simulink model "arch_logical"  (R2023b)
settings: Solver=VariableStepAuto  StartTime=0.0  StopTime=2  RelTol=1e-3
model workspace (MAT data in the model file):
  pendulum_type = Simulink.Parameter
  pendulum_type.Value = 1
  pendulum_type.DataType = 'uint8'
  pendulum_type.DocUnits = '1'
  pendulum_type.Complexity = 'real'
  pendulum_type.Dimensions = [1 1]
undefined symbols (not defined in the file): pendulum_mass
settings Model: DataDictionary=data_interface.sldd  Creator=upattacini  LastModifiedBy=upattacini
settings DataIOCC: SaveOutput=off  DSMLogging=off  SaveTime=off  ReturnWorkspaceOutputs=off
settings ModelReferenceCC: ModelReferenceNumInstancesAllowed=Single
settings ExplorerConfigSet: SimMechanicsOpenEditorOnUpdate=off  InternalSimMechanicsExplorerSettings="<ExplorerConfiguration><canonicalview>default</canonicalview><AnimationSetting><BasePlaybackSpeed>1.0</BasePlaybackSpeed><PlaybackSpeedFactor>1.0</PlaybackSpeedFactor></AnimationSetting><TilePanel><TileInfo><Tiles Columns=\"1\" Count=\"1\" Rows=\"1\"><Column Weight=\"1\"/><Row Weight=\"1\"/><Tile Height=\"1\" Width=\"1\" X=\"0\" Y=\"0\"/></Tiles></TileInfo><SceneInfo><SceneViewer><BGColor><R>0.60000002384185791</R><G>0.60000002384185791</G><B>0.60000002384185791</B></BGColor><Camera><DoPerspective>off</DoPerspective><Position><X>-0.00879418750464690258</X><Y>0.0179244290375060247</Y><Z>1.00000000042813264</Z></Position><Center><X>-0.00879418750464690258</X><Y>0.0179244290375060247</Y><Z>4.28132640450940016e-10</Z></Center><Up><X>0</X><Y>1</Y><Z>-0</Z></Up><ViewLimDist>1</ViewLimDist><YLim>0.258153931099697476</YLim><XLim>0.345051321440949021</XLim></Camera></SceneViewer></SceneInfo></TilePanel><MechEditorPanel><Cameras/><GfxPanelCameraMap/><VideoCreator><PlaybackSpeedRatio>1.0</PlaybackSpeedRatio><FrameRate>30</FrameRate><VideoFormat>Motion JPEG AVI</VideoFormat><FrameSize>auto</FrameSize></VideoCreator></MechEditorPanel></ExplorerConfiguration>"

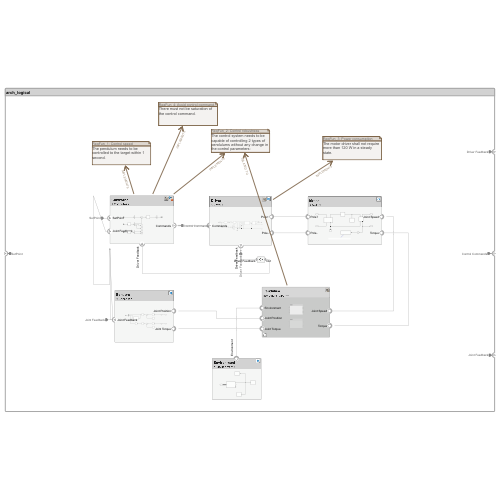
[thumbnail: Simulink's stored preview of the top-level diagram]
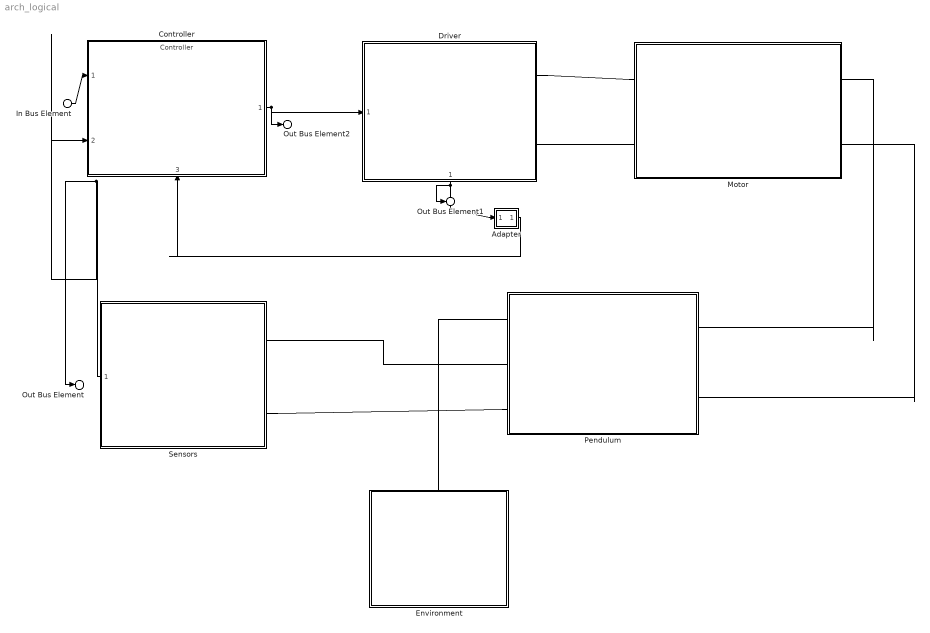
== system arch_logical ==
  In Bus Element : Inport  PortName=SetPoint
  Adapter : Subsystem
      settings: PortSchema="{\"entries\":[{\"content\":{\"margin\":10,\"minimumSpacing\":15,\"sides\":[{\"content\":{\"connectorIds\":[\"In1\"]},\"type\":\"ConnectorPlacement.EquallySpacedRectSide\",\"uuid\":\"71c09ee4-bd5d-4849-9770-0bb167b66dd4\"},{\"content\":{\"connectorIds\":[\"Out1\"],\"side\":\"RIGHT\"},\"type\":\"ConnectorPlacement.EquallySpacedRectSide\",\"uuid\":\"3c6482b7-7dc2-4555-8349-1ada307188c7\"},{\"content\":{\"side\":\"TOP\"},\"type\":\"ConnectorPlacement.EquallySpacedRectSide\",\"uuid\":\"1ceef67c-8610-4005-8087-2f0234552c2e\"}]},\"type\":\"ConnectorPlacement.EquallySpacedConnector\",\"uuid\":\"27bb57db-ed53-47ec-ba16-e40a00874efd\"}],\"packageUris\":[\"http://schema.mathworks.com/mf0/Connector/R2020b\"],\"version\":\"1.0\"}"
  Controller : ModelReference  ModelNameDialog=Controller  SimulationMode=Normal  ModelReferenceVersion=1.47
      settings: PortSchema="{\"entries\":[{\"content\":{\"headerSize\":38,\"margin\":15,\"minimumSpacing\":25,\"sides\":[{\"content\":{\"connectorIds\":[\"In1\",\"In2\"]},\"type\":\"ConnectorPlacement.EquallySpacedRectSide\",\"uuid\":\"cda6e8c3-28ef-478a-8903-19efeda1d005\"},{\"content\":{\"connectorIds\":[\"Out1\"],\"side\":\"RIGHT\"},\"type\":\"ConnectorPlacement.EquallySpacedRectSide\",\"uuid\":\"ea374fb9-fe28-40dc-ac3e-322c9df25f40\"},{\"content\":{\"side\":\"TOP\"},\"type\":\"ConnectorPlacement.EquallySpacedRectSide\",\"uuid\":\"d8bce015-985d-440b-ab42-a24854ac657a\"},{\"content\":{\"connectorIds\":[\"In3\"],\"side\":\"BOTTOM\"},\"type\":\"ConnectorPlacement.EquallySpacedRectSide\",\"uuid\":\"ef4904ce-87a8-4dd7-afa5-50688cfaf5d0\"}]},\"type\":\"ConnectorPlacement.EquallySpacedConnector\",\"uuid\":\"3fae5f3d-400e-4110-946e-917d26d89769\"}],\"packageUris\":[\"http://schema.mathworks.com/mf0/Connector/R2020b\"],\"version\":\"1.0\"}"
  Driver : Subsystem  ReferencedSubsystem=Driver
      settings: PermitHierarchicalResolution=None  PortSchema="{\"entries\":[{\"content\":{\"headerSize\":26,\"margin\":15,\"minimumSpacing\":25,\"sides\":[{\"content\":{\"connectorIds\":[\"In1\"]},\"type\":\"ConnectorPlacement.EquallySpacedRectSide\",\"uuid\":\"87b13320-d2be-495c-9e0a-d50be08d4455\"},{\"content\":{\"connectorIds\":[\"RConn1\",\"RConn2\"],\"side\":\"RIGHT\"},\"type\":\"ConnectorPlacement.EquallySpacedRectSide\",\"uuid\":\"602bd151-4107-439e-8200-46b9490e5c42\"},{\"content\":{\"side\":\"TOP\"},\"type\":\"ConnectorPlacement.EquallySpacedRectSide\",\"uuid\":\"a9c961f8-1e8e-4fd0-91ed-15da0975152b\"},{\"content\":{\"connectorIds\":[\"Out1\"],\"side\":\"BOTTOM\"},\"type\":\"ConnectorPlacement.EquallySpacedRectSide\",\"uuid\":\"ffc1b1ec-88d8-4f39-9e46-3aab7c832f5b\"}]},\"type\":\"ConnectorPlacement.EquallySpacedConnector\",\"uuid\":\"8c5d9a44-25d8-4d3b-8680-514fbe3d26a8\"}],\"packageUris\":[\"http://schema.mathworks.com/mf0/Connector/R2020b\"],\"version\":\"1.0\"}"
  Environment : Subsystem  ReferencedSubsystem=Environment
      settings: PermitHierarchicalResolution=None  PortSchema="{\"entries\":[{\"content\":{\"headerSize\":26,\"margin\":15,\"minimumSpacing\":25,\"sides\":[{\"content\":{},\"type\":\"ConnectorPlacement.EquallySpacedRectSide\",\"uuid\":\"45a2255a-b64b-4ce6-b48f-d923e11d651c\"},{\"content\":{\"side\":\"RIGHT\"},\"type\":\"ConnectorPlacement.EquallySpacedRectSide\",\"uuid\":\"23c27b1d-8e45-436e-af19-695457c59d8d\"},{\"content\":{\"connectorIds\":[\"LConn1\"],\"side\":\"TOP\"},\"type\":\"ConnectorPlacement.EquallySpacedRectSide\",\"uuid\":\"da7f94f3-b927-4bf7-a124-148f2fc7ec34\"}]},\"type\":\"ConnectorPlacement.EquallySpacedConnector\",\"uuid\":\"db435fa4-4dbe-4289-bd60-c3db6d84fa67\"}],\"packageUris\":[\"http://schema.mathworks.com/mf0/Connector/R2020b\"],\"version\":\"1.0\"}"
  Motor : Subsystem  ReferencedSubsystem=Motor
      settings: PermitHierarchicalResolution=None  PortSchema="{\"entries\":[{\"content\":{\"headerSize\":26,\"margin\":15,\"minimumSpacing\":25,\"sides\":[{\"content\":{\"connectorIds\":[\"LConn1\",\"LConn2\"]},\"type\":\"ConnectorPlacement.EquallySpacedRectSide\",\"uuid\":\"cda6e8c3-28ef-478a-8903-19efeda1d005\"},{\"content\":{\"connectorIds\":[\"RConn1\",\"RConn2\"],\"side\":\"RIGHT\"},\"type\":\"ConnectorPlacement.EquallySpacedRectSide\",\"uuid\":\"ea374fb9-fe28-40dc-ac3e-322c9df25f40\"},{\"content\":{\"side\":\"TOP\"},\"type\":\"ConnectorPlacement.EquallySpacedRectSide\",\"uuid\":\"d8bce015-985d-440b-ab42-a24854ac657a\"}]},\"type\":\"ConnectorPlacement.EquallySpacedConnector\",\"uuid\":\"3fae5f3d-400e-4110-946e-917d26d89769\"}],\"packageUris\":[\"http://schema.mathworks.com/mf0/Connector/R2020b\"],\"version\":\"1.0\"}"
  Pendulum : Subsystem  Variant=on
      settings: PortSchema="{\"entries\":[{\"content\":{\"headerSize\":38,\"margin\":15,\"minimumSpacing\":25,\"sides\":[{\"content\":{\"connectorIds\":[\"LConn1\",\"LConn2\",\"LConn3\"]},\"type\":\"ConnectorPlacement.EquallySpacedRectSide\",\"uuid\":\"bf58af0e-2227-4325-b7b4-ca7aa5d9b389\"},{\"content\":{\"connectorIds\":[\"RConn1\",\"RConn2\"],\"side\":\"RIGHT\"},\"type\":\"ConnectorPlacement.EquallySpacedRectSide\",\"uuid\":\"91e52710-35d3-4d9b-803d-8a6447c25190\"},{\"content\":{\"side\":\"TOP\"},\"type\":\"ConnectorPlacement.EquallySpacedRectSide\",\"uuid\":\"a9a735dd-f81f-408b-81bc-2d8dc361c4fb\"}]},\"type\":\"ConnectorPlacement.EquallySpacedConnector\",\"uuid\":\"4c4e0bb0-440d-47ff-82c5-294788dc91eb\"}],\"packageUris\":[\"http://schema.mathworks.com/mf0/Connector/R2020b\"],\"version\":\"1.0\"}"
  Sensors : Subsystem  ReferencedSubsystem=Sensors
      settings: PermitHierarchicalResolution=None  PortSchema="{\"entries\":[{\"content\":{\"headerSize\":26,\"margin\":15,\"minimumSpacing\":25,\"sides\":[{\"content\":{\"connectorIds\":[\"Out1\"]},\"type\":\"ConnectorPlacement.EquallySpacedRectSide\",\"uuid\":\"45a2255a-b64b-4ce6-b48f-d923e11d651c\"},{\"content\":{\"connectorIds\":[\"RConn1\",\"RConn2\"],\"side\":\"RIGHT\"},\"type\":\"ConnectorPlacement.EquallySpacedRectSide\",\"uuid\":\"23c27b1d-8e45-436e-af19-695457c59d8d\"},{\"content\":{\"side\":\"TOP\"},\"type\":\"ConnectorPlacement.EquallySpacedRectSide\",\"uuid\":\"da7f94f3-b927-4bf7-a124-148f2fc7ec34\"}]},\"type\":\"ConnectorPlacement.EquallySpacedConnector\",\"uuid\":\"db435fa4-4dbe-4289-bd60-c3db6d84fa67\"}],\"packageUris\":[\"http://schema.mathworks.com/mf0/Connector/R2020b\"],\"version\":\"1.0\"}"
  Out Bus Element1 : Outport  PortName=Driver Feedback
  Out Bus Element2 : Outport  Port=2  PortName=Control Commands
  Out Bus Element : Outport  Port=3  PortName=Joint Feedback
  wires:
  Sensors/1 -> Out Bus Element/1, Controller/2
  Driver/1 -> Out Bus Element1/1, Adapter/1(Driver Feedback)
  In Bus Element/1 -> Controller/1
  Controller/1 -> Out Bus Element2/1, Driver/1
  Adapter/1(Out) -> Controller/3
  connections:
  Driver/RConn2 -- Motor/LConn2
  Driver/RConn1 -- Motor/LConn1
  Motor/RConn1 -- Pendulum/RConn1
  Motor/RConn2 -- Pendulum/RConn2
  Environment/LConn1 -- Pendulum/LConn1
  Sensors/RConn1 -- Pendulum/LConn2
  Sensors/RConn2 -- Pendulum/LConn3

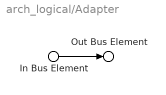
== system arch_logical/Adapter ==
  In Bus Element : Inport  PortName=Driver Feedback
  Out Bus Element : Outport  PortName=Out
  wires:
  In Bus Element/1 -> Out Bus Element/1

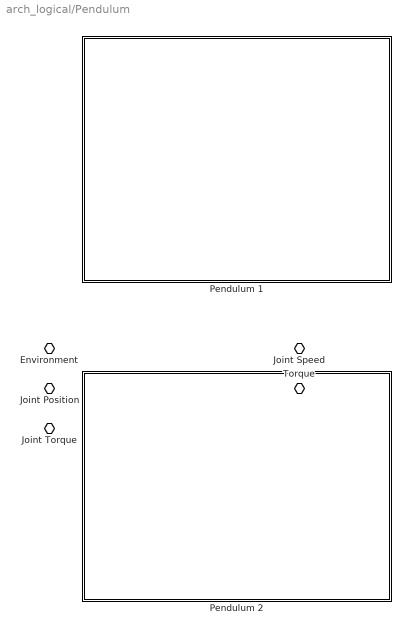
== system arch_logical/Pendulum ==
  Pendulum 1 : Subsystem  VariantControl=pendulum_type == 1  ReferencedSubsystem=Pendulum  l=pendulum_1_length  m=pendulum_mass
      settings: PermitHierarchicalResolution=None  PortSchema="{\"entries\":[{\"content\":{\"headerSize\":26,\"margin\":15,\"minimumSpacing\":25,\"sides\":[{\"content\":{\"connectorIds\":[\"LConn1\",\"LConn2\",\"LConn3\"]},\"type\":\"ConnectorPlacement.EquallySpacedRectSide\",\"uuid\":\"82f5cb4d-4a78-40c4-a21e-410695f42653\"},{\"content\":{\"connectorIds\":[\"RConn1\",\"RConn2\"],\"side\":\"RIGHT\"},\"type\":\"ConnectorPlacement.EquallySpacedRectSide\",\"uuid\":\"035de433-2e3e-4321-a7d9-a74f0d831365\"},{\"content\":{\"side\":\"TOP\"},\"type\":\"ConnectorPlacement.EquallySpacedRectSide\",\"uuid\":\"ce921c4a-a98b-4acd-b6b2-e0e0d1283243\"}]},\"type\":\"ConnectorPlacement.EquallySpacedConnector\",\"uuid\":\"03220c26-1eff-4576-b7d6-6d5cd293b475\"}],\"packageUris\":[\"http://schema.mathworks.com/mf0/Connector/R2020b\"],\"version\":\"1.0\"}"
  Pendulum 2 : Subsystem  VariantControl=pendulum_type == 2  ReferencedSubsystem=Pendulum  l=pendulum_2_length  m=pendulum_mass
      settings: PermitHierarchicalResolution=None  PortSchema="{\"entries\":[{\"content\":{\"headerSize\":26,\"margin\":15,\"minimumSpacing\":25,\"sides\":[{\"content\":{\"connectorIds\":[\"LConn1\",\"LConn2\",\"LConn3\"]},\"type\":\"ConnectorPlacement.EquallySpacedRectSide\",\"uuid\":\"82f5cb4d-4a78-40c4-a21e-410695f42653\"},{\"content\":{\"connectorIds\":[\"RConn1\",\"RConn2\"],\"side\":\"RIGHT\"},\"type\":\"ConnectorPlacement.EquallySpacedRectSide\",\"uuid\":\"035de433-2e3e-4321-a7d9-a74f0d831365\"},{\"content\":{\"side\":\"TOP\"},\"type\":\"ConnectorPlacement.EquallySpacedRectSide\",\"uuid\":\"ce921c4a-a98b-4acd-b6b2-e0e0d1283243\"}]},\"type\":\"ConnectorPlacement.EquallySpacedConnector\",\"uuid\":\"03220c26-1eff-4576-b7d6-6d5cd293b475\"}],\"packageUris\":[\"http://schema.mathworks.com/mf0/Connector/R2020b\"],\"version\":\"1.0\"}"
  Joint Speed : PMIOPort  Side=Right
  Torque : PMIOPort  Port=2  Side=Right
  Environment : PMIOPort  Port=3  Side=Left
  Joint Position : PMIOPort  Port=4  Side=Left
  Joint Torque : PMIOPort  Port=5  Side=Left
